simulink model "Rotpentemplate_down_down_PID_FINAL"  (R2020b)
settings: Solver=ode45  StartTime=0.0  StopTime=60  RelTol=1e-3  EnableMultiTasking=on
values from neighbouring files (symbols this model uses):
  g01 = mean_data(2)    [MainScript_PID.m]    (also in calib_up_up.m)
  g02 = mean_data(3)    [MainScript_PID.m]    (also in calib_up_up.m)
  g11 = (mean_data(2)-mean_data(1))/pi    [MainScript_PID.m]    (also in calib_up_up.m)
  g12 = (mean_data(3)-mean_data(4))/pi    [MainScript_PID.m]    (also in calib_up_up.m)
  h = 0.01    [MainScript_PID.m]    (also in calib_up_up.m = 0.005)
undefined symbols (not defined in the file or in its folder): adingain, adinoffs, daoutgain, daoutoffs
libraries: dspsigops x2, pid_lib x1
settings Model: Creator=rbabuska  LastModifiedBy=llaporte
settings DataIOCC: LimitDataPoints=on  SaveFormat=Array  ReturnWorkspaceOutputs=off  SignalLoggingName=sigsOut
settings OptimizationCC: BooleanDataType=off  ExpressionDepthLimit=2147483647  InitFltsAndDblsToZero=on  LifeSpan=inf
settings DebuggingCC: SaveWithParameterizedLinksMsg=none  SignalResolutionControl=TryResolveAllWithWarning  MultiTaskDSMMsg=warning  MultiTaskCondExecSysMsg=none  AllowSymbolicDim=off  StateNameClashWarn=warning  SFUnexpectedBacktrackingDiag=warning  SFNoUnconditionalDefaultTransitionDiag=warning  SFExecutionAtInitializationDiag=none  ArithmeticOperatorsInVariantConditions=warning
settings HardwareCC: ProdBitPerPointer=32  ProdBitPerSizeT=32  ProdBitPerPtrDiffT=32  ProdLargestAtomicFloat=None  ProdIntDivRoundTo=Undefined  ProdEndianess=Unspecified  ProdWordSize=32  ProdHWDeviceType=32-bit Generic  TargetUnknown=on
settings ModelReferenceCC: PropagateSignalLabelsOutOfModel=off
settings SFSimCC: SimUseLocalCustomCode=off  CustomCodeUndefinedFunction=UseInterfaceOnly
settings RTWCC: RTWUseLocalCustomCode=off
settings CodeAppCC: StateflowObjectComments=on
settings GRTTargetCC: TargetFcnLib=ansi_tfl_tmw.mat  TargetLangStandard=C89/C90 (ANSI)  CombineOutputUpdateFcns=off  GRTInterface=on
settings ConfigComp: CovMetricSettings=dw  CovSaveCumulativeToWorkspaceVar=on  CovSaveSingleToWorkspaceVar=on  CovExternalEMLEnable=off

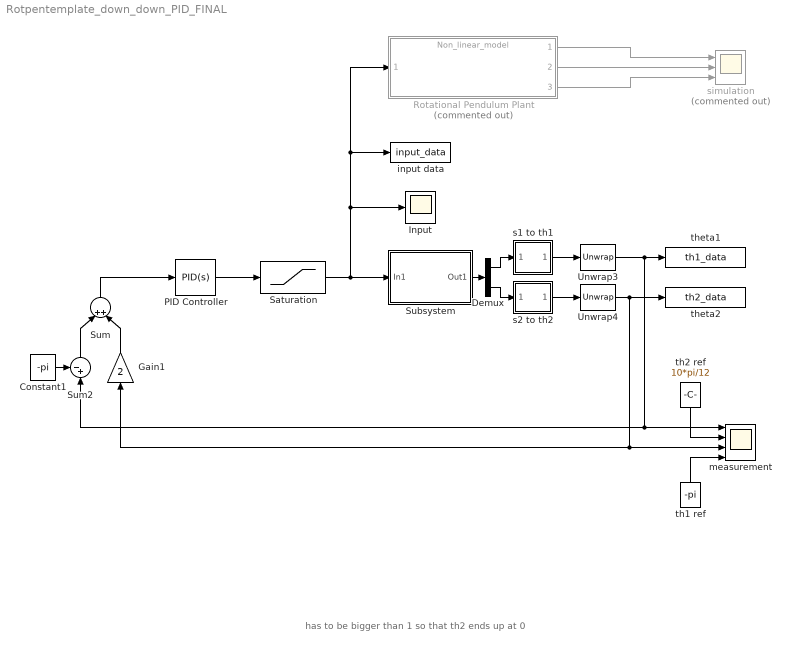
== system Rotpentemplate_down_down_PID_FINAL ==
  note: has to be bigger than 1 so that th2 ends up at 0
  Constant1 : Constant  Value=-pi
  Demux : Demux  Outputs=2
  Gain1 : Gain  Gain=2
  Input : Scope
  PID Controller : pid_lib/PID Controller  Controller=PID  Form=Parallel  TimeDomain=Continuous-time  UseExternalTs=off  SampleTime=-1  IntegratorMethod=Forward Euler  FilterMethod=Forward Euler  ControllerParametersSource=internal  P=1  I=0  D=-0.4  UseFilter=on  N=1  TunerSelectOption=Transfer Function Based (PID Tuner App)  InitialConditionSource=internal  InitialConditionForIntegrator=0  InitialConditionForFilter=0  DifferentiatorICPrevScaledInput=0  ExternalReset=none  TrackingMode=off  Kt=1  LimitOutput=off  SatLimitsSource=internal  UpperSaturationLimit=inf  LowerSaturationLimit=-inf  LinearizeAsGain=on  AntiWindupMode=none  Kb=1  POutMin=[]  POutMax=[]  IOutMin=[]  IOutMax=[]  DOutMin=[]  DOutMax=[]  NOutMin=[]  NOutMax=[]  SumOutMin=[]  SumOutMax=[]  SaturationOutMin=[]  SaturationOutMax=[]  PParamMin=[]  PParamMax=[]  IParamMin=[]  IParamMax=[]  DParamMin=[]  DParamMax=[]  NParamMin=[]  NParamMax=[]  KbParamMin=[]  KbParamMax=[]  KtParamMin=[]  KtParamMax=[]  KbOutMin=[]  KbOutMax=[]  KtOutMin=[]  KtOutMax=[]  IntegratorOutMin=[]  IntegratorOutMax=[]  FilterOutMin=[]  FilterOutMax=[]  SumI1OutMin=[]  SumI1OutMax=[]  SumI2OutMin=[]  SumI2OutMax=[]  SumI3OutMin=[]  SumI3OutMax=[]  SumI4OutMin=[]  SumI4OutMax=[]  SumDOutMin=[]  SumDOutMax=[]  DifferentiatorOutMin=[]  DifferentiatorOutMax=[]  FilterDiffOutCoefMin=[]  FilterDiffOutCoefMax=[]  ReciprocalOutMin=[]  ReciprocalOutMax=[]  SumDenOutMin=[]  SumDenOutMax=[]  SumNumOutMin=[]  SumNumOutMax=[]  DivideOutMin=[]  DivideOutMax=[]  UdiffTsProdOutMin=[]  UdiffTsProdOutMax=[]  NTsProdOutMin=[]  NTsProdOutMax=[]  UintegralTsProdOutMin=[]  UintegralTsProdOutMax=[]  UngainTsProdOutMin=[]  UngainTsProdOutMax=[]  IntegratorContinuousStateAttributes=''  IntegratorStateMustResolveToSignalObject=off  IntegratorRTWStateStorageClass=Auto  FilterContinuousStateAttributes=''  FilterStateMustResolveToSignalObject=off  FilterRTWStateStorageClass=Auto  ParallelPVariant=InternalParameters  IdealPVariant=Disabled  IVariant=InternalParameters  DVariant=InternalParameters  IntegratorVariant=Continuous  SatVariant=Disabled  AWVariant=Passthrough  PCopyVariant=Disabled  TRVariant=Disabled  FdbkBlocksVariant=Forward  IdealPFdbkVariant=Disabled  SatFdbkVariant=Disabled  DerivativeFilterVariant=ContFilter  NVariant=InternalParameters  NCopyVariant=Disabled  FilterICVariant=InternalICsFilter  IntegratorICVariant=InternalICs  ExternalResetVariant=Disabled  TRSumVariant=Passthrough  SumFdbkVariant=Disabled  SumVariant=Sum_PID  TsampFilterVariant=InternalTs  TsampNgainVariant=Passthrough  TsampIntegralVariant=Passthrough  ExternalSaturationOutDataTypeStr=Inherit: Same as second input
  Rotational Pendulum Plant : ModelReference  Commented=on  ModelNameDialog=Non_linear_model.slx  SimulationMode=Normal  ModelReferenceVersion=3.13
  Saturation : Saturate  UpperLimit=1  LowerLimit=-1
  Subsystem : Subsystem
      mask Display: disp('Rotational\nPendulum')
  Sum : Sum  Inputs=|++|
  Sum2 : Sum  Inputs=-+|
  Unwrap3 : dspsigops/Unwrap  tol=pi  InputProcessing=Columns as channels (frame based)  running=off
  Unwrap4 : dspsigops/Unwrap  tol=pi  InputProcessing=Columns as channels (frame based)  running=off
  input data : ToWorkspace  VariableName=input_data  SaveFormat=Timeseries  SampleTime=h
  measurement : Scope  NumInputPorts=4
  s1 to th1 : Subsystem
  s2 to th2 : Subsystem
  simulation : Scope  Commented=on  NumInputPorts=3
  th1 ref : Constant  Value=-pi
  th2 ref : Constant  Value=10*pi/12
  theta1 : ToWorkspace  VariableName=th1_data  SaveFormat=Timeseries  SampleTime=h
  theta2 : ToWorkspace  VariableName=th2_data  SaveFormat=Timeseries  SampleTime=h
  wires:
  Saturation/1 -> Subsystem/1(In1), Input/1, input data/1, Rotational Pendulum Plant/1
  Subsystem/1(Out1) -> Demux/1
  Demux/1 -> s1 to th1/1(v1)
  Demux/2 -> s2 to th2/1(v2)
  Rotational Pendulum Plant/1 -> simulation/1
  Rotational Pendulum Plant/2 -> simulation/2
  Rotational Pendulum Plant/3 -> simulation/3
  s1 to th1/1(th1) -> Unwrap3/1
  Unwrap3/1 -> Sum2/2, measurement/1, theta1/1
  s2 to th2/1(th2) -> Unwrap4/1
  th1 ref/1 -> measurement/4
  th2 ref/1 -> measurement/2
  PID Controller/1 -> Saturation/1
  Constant1/1 -> Sum2/1
  Unwrap4/1 -> Gain1/1, measurement/3, theta2/1
  Gain1/1 -> Sum/2
  Sum/1 -> PID Controller/1
  Sum2/1 -> Sum/1

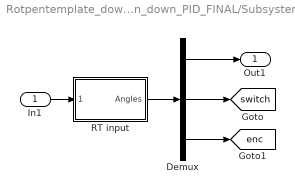
== system Rotpentemplate_down_down_PID_FINAL/Subsystem ==
  In1 : Inport
  Demux : Demux  Outputs=[2 4 1]
  RT input : Subsystem  mask{Ts=h, channels=[6 7]}
      mask prompts: Ts "Sample time [s]:"; channels "Channels to read (e.g., [6 7])"
      mask init:
      | hwinit;
      | 
      | % initialize FPGA
      | fugihandle = fugiboard('Open', 'Pendulum1');
      | fugihandle.WatchdogTimeout = 0.5;
      | fugiboard('SetParams', fugihandle);
      | fugiboard('Write', fugihandle, 0, 0, 0, 0);  % dummy write to sync interface board
      | fugiboard('Write', fugihandle, 5, 1, 0, 0);  % reset position, activate relay
      | data = fugiboard('Read', fugihandle);        % get version info from FPGA
      | % model = bitshift(data(1), -5); 
      | % version = bitand(data(1), 31);
      | % disp(sprintf('FPGA setup %d, version %d', model, version)); % for the B&P it should say 1 1, or else there is a problem
      | fugiboard('Write', fugihandle, 0, 1, 0, 0);  % end reset
      | pause(0.1);                         % give relay some time to respond
      mask Display: disp('Rotational\nPendulum')
  Out1 : Outport
  tag scope: enc=global, switch=global
  wires:
  RT input/1(Angles) -> Demux/1
  Demux/1 -> Out1/1
  Demux/2 -> [switch]
  Demux/3 -> [enc]
  In1/1 -> RT input/1(Motors)

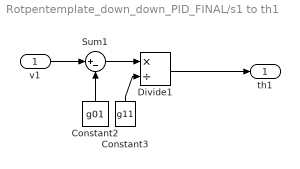
== system Rotpentemplate_down_down_PID_FINAL/s1 to th1 ==
  v1 : Inport
  Constant2 : Constant  Value=g01
  Constant3 : Constant  Value=g11
  Divide1 : Product  Inputs=*/
  Sum1 : Sum  Inputs=|+-
  th1 : Outport
  wires:
  Constant2/1 -> Sum1/2
  Constant3/1 -> Divide1/2
  Divide1/1 -> th1/1
  Sum1/1 -> Divide1/1
  v1/1 -> Sum1/1

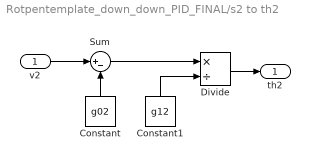
== system Rotpentemplate_down_down_PID_FINAL/s2 to th2 ==
  v2 : Inport
  Constant : Constant  Value=g02
  Constant1 : Constant  Value=g12
  Divide : Product  Inputs=*/
  Sum : Sum  Inputs=|+-
  th2 : Outport
  wires:
  Constant1/1 -> Divide/2
  Divide/1 -> th2/1
  Constant/1 -> Sum/2
  Sum/1 -> Divide/1
  v2/1 -> Sum/1

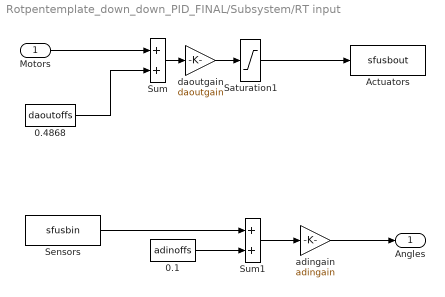
== system Rotpentemplate_down_down_PID_FINAL/Subsystem/RT input ==
  Motors : Inport
  0.1 : Constant  Value=adinoffs
  0.4868 : Constant  Value=daoutoffs
  Actuators : S-Function  FunctionName=sfusbout  Parameters=Ts, fugihandle  SFunctionDeploymentMode=off  EnableBusSupport=off
  Saturation1 : Saturate  UpperLimit=10  LowerLimit=-10
  Sensors : S-Function  FunctionName=sfusbin  Parameters=Ts, fugihandle, channels  SFunctionDeploymentMode=off  EnableBusSupport=off
  Sum : Sum  InputSameDT=on  SaturateOnIntegerOverflow=on  OutDataTypeStr=Inherit: Same as first input
  Sum1 : Sum  InputSameDT=on  SaturateOnIntegerOverflow=on  OutDataTypeStr=Inherit: Same as first input
  adingain : Gain  Gain=adingain  SaturateOnIntegerOverflow=on  OutDataTypeStr=Inherit: Same as input  ParamDataTypeStr=Inherit: Same as input
  daoutgain : Gain  Gain=daoutgain  SaturateOnIntegerOverflow=on  OutDataTypeStr=Inherit: Same as input  ParamDataTypeStr=Inherit: Same as input
  Angles : Outport
  wires:
  Sum/1 -> daoutgain/1
  0.4868/1 -> Sum/2
  Motors/1 -> Sum/1
  Sum1/1 -> adingain/1
  0.1/1 -> Sum1/2
  adingain/1 -> Angles/1
  Saturation1/1 -> Actuators/1
  daoutgain/1 -> Saturation1/1
  Sensors/1 -> Sum1/1
